simulink model "OL_Step_Resp_Arduino"  (R2016b)
settings: Solver=FixedStepDiscrete  StartTime=0.0  StopTime=inf  FixedStep=Ts  RelTol=1e-3  EnableMultiTasking=on
InitFcn:
  | Ts = 0.01;
  | rp = 2*pi/1336;
libraries: arduinolib x2, THLlib x2, simulink x1
settings Model: ExtModeTrigDuration=2  Creator=Carion  LastModifiedBy=maeuser
settings DataIOCC: LimitDataPoints=on  SaveFormat=Array
settings OptimizationCC: MaxStackSize=64
settings DebuggingCC: UnderspecifiedInitializationDetection=Classic  MergeDetectMultiDrivingBlocksExec=none  ParameterTunabilityLossMsg=error  StateNameClashWarn=warning  SFUnexpectedBacktrackingDiag=warning  SFNoUnconditionalDefaultTransitionDiag=warning  SFExecutionAtInitializationDiag=none
settings HardwareCC: ProdBitPerInt=16  ProdBitPerPointer=16  ProdBitPerSizeT=16  ProdBitPerPtrDiffT=16  ProdLargestAtomicFloat=None  ProdWordSize=8  ProdHWDeviceType=Atmel->AVR
settings ModelReferenceCC: PropagateSignalLabelsOutOfModel=off
settings RTWCC: SystemTargetFile=ert.tlc  HardwareBoard=Arduino Mega 2560  TLCOptions=-aInlineSetEventsForThisBaseRateFcn=TLC_FALSE -aSuppressMultiTaskScheduler=TLC_FALSE -aRateBasedStepFcn=1  TemplateMakefile=ert_default_tmf  Description=Embedded Coder  GenerateReport=on  RTWVerbose=off  Toolchain=Arduino AVR  BuildConfiguration=Faster Runs  IncludeHyperlinkInReport=on  LaunchReport=on  GenerateTraceInfo=on  GenerateTraceReport=on  GenerateTraceReportSl=on  GenerateTraceReportSf=on  GenerateTraceReportEml=on
settings CodeAppCC: ForceParamTrailComments=on  IgnoreCustomStorageClasses=off  OperatorAnnotations=on  SimulinkDataObjDesc=on  SFDataObjDesc=on  MATLABFcnDesc=on  InsertBlockDesc=on  MATLABSourceComments=on
settings ERTTargetCC: SupportContinuousTime=on  SupportVariableSizeSignals=on
settings ConfigComp: CovMetricSettings=dw  CovHtmlReporting=on  CovSaveCumulativeToWorkspaceVar=on  CovSaveSingleToWorkspaceVar=on  CovExternalEMLEnable=off

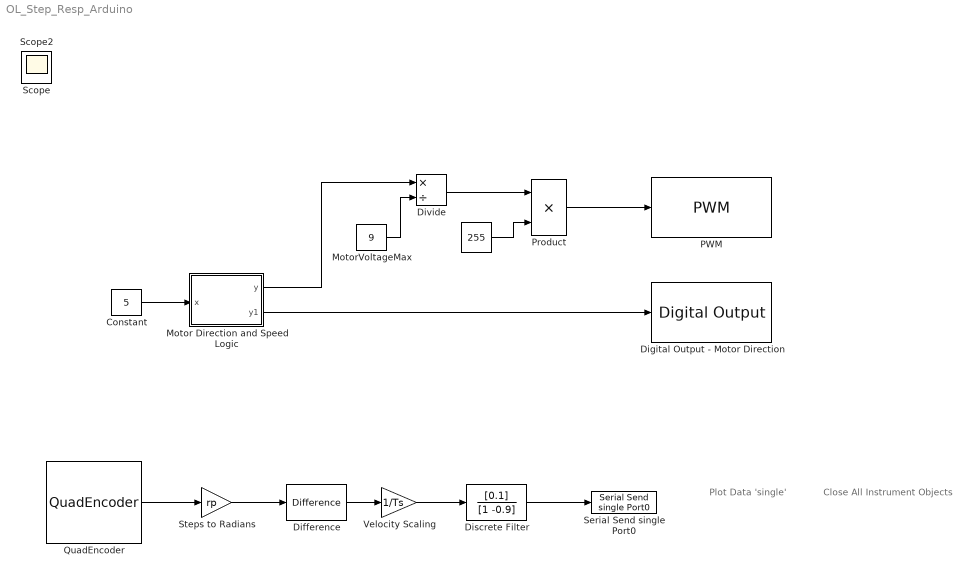
== system OL_Step_Resp_Arduino ==
  note: Close All
      | Instrument Objects
  note: Plot Data
      | 'single'
  " " : Constant  Value=255  SampleTime=Ts
  Constant : Constant  Value=5  SampleTime=Ts
  Difference : simulink/Discrete/Difference  ICPrevInput=0.0  InputProcessing=Inherited  OutMin=[]  OutMax=[]  OutDataType=fixdt(1, 16)  OutScaling=2^-10  DoSatur=off
  Digital Output - Motor Direction : arduinolib/Digital Output  pinNumber=4  blockPlatform=arduino
  Discrete Filter : DiscreteFilter  Numerator=[0.1]  Denominator=[1 -0.9]  SampleTime=Ts
  Divide : Product  Inputs=*/  SampleTime=Ts
  Motor Direction and Speed Logic : MATLAB Function  TreatAsAtomicUnit=on
  MotorVoltageMax : Constant  Value=9  SampleTime=Ts
  PWM : arduinolib/PWM  pinNumber=5  blockPlatform=arduino
  Product : Product  SampleTime=Ts
  QuadEncoder : THLlib/QuadEncoder
  Serial Send single Port0 : THLlib/Serial Send single Port0
  Steps to Radians : Gain  Gain=rp
  Velocity Scaling : Gain  Gain=1/Ts
  Scope : Scope
  Scope2 : Scope
  wires:
  " "/1 -> Product/2
  Product/1 -> PWM/1
  MotorVoltageMax/1 -> Divide/2
  Divide/1 -> Product/1
  Motor Direction and Speed Logic/2(y1) -> Digital Output - Motor Direction/1
  Constant/1 -> Motor Direction and Speed Logic/1(x)
  Motor Direction and Speed Logic/1(y) -> Divide/1
  QuadEncoder/1 -> Steps to Radians/1
  Steps to Radians/1 -> Difference/1
  Difference/1 -> Velocity Scaling/1
  Velocity Scaling/1 -> Discrete Filter/1
  Discrete Filter/1 -> Serial Send single Port0/1

== matlab function OL_Step_Resp_Arduino/Motor Direction and Speed Logic ==
  data: x input; y output; y1 output
function [y,y1] = fcn(x)
%#codegen
if x>=0
    y=x;
    y1=0;
else
    y=-x;
    y1=1;
end
